simulink model "linear_closed_loop"  (R2025b)
settings: Solver=VariableStepAuto  StartTime=0.0  StopTime=200  RelTol=1e-3
undefined symbols (not defined in the file or in its folder): ra, rw, SATP
libraries: simulink_extras x2, cstblocks x1
settings Model: Creator=ruben  LastModifiedBy=flori

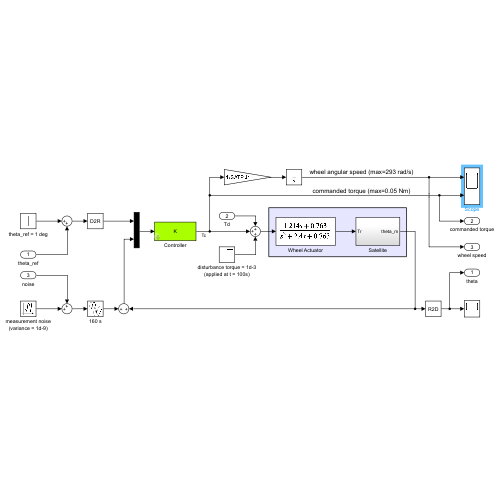
[thumbnail: Simulink's stored preview of the top-level diagram]
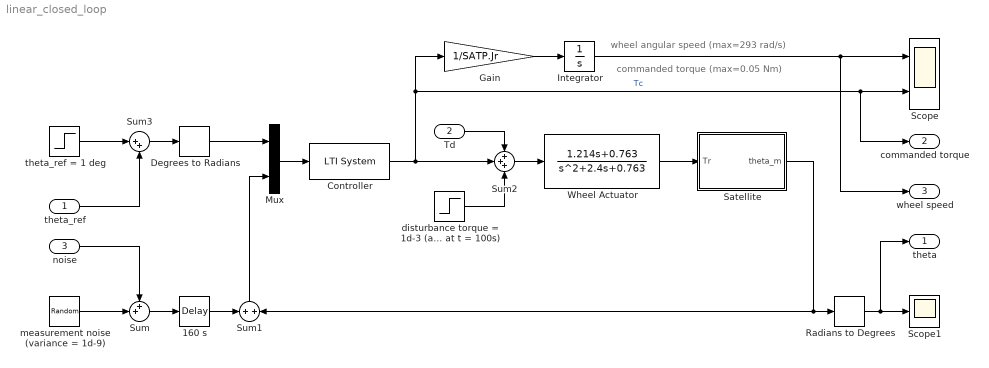
== system linear_closed_loop ==
  note: commanded torque (max=0.05 Nm)
  note: wheel angular speed (max=293 rad/s)
  theta_ref : Inport
  Td : Inport  Port=2
  noise : Inport  Port=3
  160 s : TransportDelay  DelayTime=160
  Controller : cstblocks/LTI System  sys=K  IC=[]  PadeOrder=0
  Degrees to Radians : simulink_extras/Transformations/Degrees to Radians
  Gain : Gain  Gain=1/SATP.Jr
  Integrator : Integrator
  Mux : Mux  Inputs=2
  Radians to Degrees : simulink_extras/Transformations/Radians to Degrees
  Satellite : Subsystem
  Scope : Scope  NumInputPorts=2
      settings: ActiveDisplayYMinimum=-302.85258313612223  ActiveDisplayYMaximum=227.5319246996597
  Scope1 : Scope
      settings: ActiveDisplayYMinimum=-0.33126841558150821  ActiveDisplayYMaximum=2.4578398850529664
  Sum : Sum  Inputs=++|
  Sum1 : Sum  Inputs=+|+
  Sum2 : Sum  Inputs=+++
  Sum3 : Sum  Inputs=|++
  Wheel Actuator : TransferFcn  Numerator=[1.214 0.763]  Denominator=[1 2.4 0.763]
  disturbance torque = 1d-3 (applied at t = 100s) : Step  Time=100  After=SATP.Td  SampleTime=0
  measurement noise (variance = 1d-9) : RandomNumber  Variance=SATP.sigmam2  SampleTime=0.01
  theta_ref = 1 deg : Step  Time=0  SampleTime=0
  theta : Outport
  commanded torque : Outport  Port=2
  wheel speed : Outport  Port=3
  wires:
  disturbance torque = 1d-3 (applied at t = 100s)/1 -> Sum2/3
  Sum/1 -> 160 s/1
  Sum2/1 -> Wheel Actuator/1
  measurement noise (variance = 1d-9)/1 -> Sum/2
  Gain/1 -> Integrator/1
  Mux/1 -> Controller/1
  Integrator/1 -> wheel speed/1, Scope/1
  theta_ref = 1 deg/1 -> Sum3/1
  noise/1 -> Sum/1
  theta_ref/1 -> Sum3/2
  160 s/1 -> Sum1/1
  Satellite/1(theta_m) -> Radians to Degrees/1, Sum1/2
  Radians to Degrees/1 -> Scope1/1, theta/1
  Degrees to Radians/1 -> Mux/1
  Td/1 -> Sum2/1
  Sum3/1 -> Degrees to Radians/1
  Sum1/1 -> Mux/2
  Controller/1 -> Sum2/2, Gain/1, Scope/2, commanded torque/1  "Tc"
  Wheel Actuator/1 -> Satellite/1(Tr)

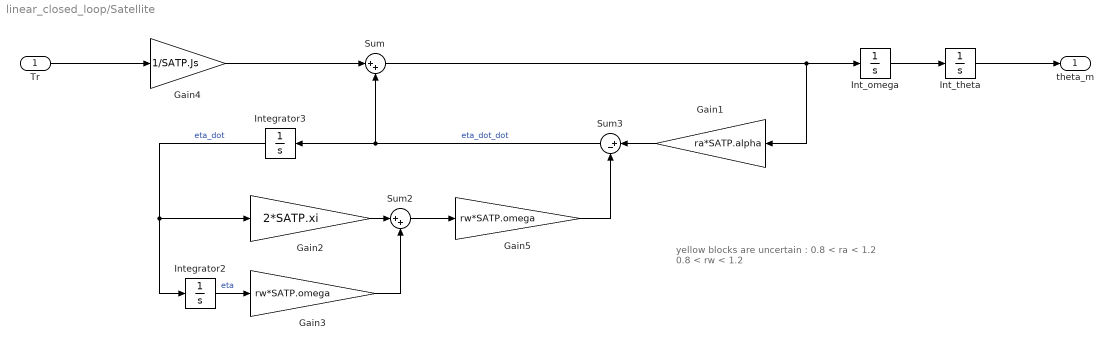
== system linear_closed_loop/Satellite ==
  note: yellow blocks are uncertain :
      | 0.8 < ra < 1.2
      | 0.8 < rw < 1.2
  Tr : Inport
  Gain1 : Gain  Gain=ra*SATP.alpha
  Gain2 : Gain  Gain=2*SATP.xi
  Gain3 : Gain  Gain=rw*SATP.omega
  Gain4 : Gain  Gain=1/SATP.Js
  Gain5 : Gain  Gain=rw*SATP.omega
  Int_omega : Integrator
  Int_theta : Integrator
  Integrator2 : Integrator  InitialCondition=SATP.eta0
  Integrator3 : Integrator
  Sum : Sum  Inputs=|++
  Sum2 : Sum  Inputs=|++
  Sum3 : Sum  Inputs=|+-
  theta_m : Outport
  wires:
  Integrator3/1 -> Integrator2/1, Gain2/1  "eta_dot"
  Int_omega/1 -> Int_theta/1
  Sum/1 -> Int_omega/1, Gain1/1
  Gain2/1 -> Sum2/1
  Gain4/1 -> Sum/1
  Gain3/1 -> Sum2/2
  Gain1/1 -> Sum3/1
  Tr/1 -> Gain4/1
  Sum3/1 -> Integrator3/1, Sum/2  "eta_dot_dot"
  Int_theta/1 -> theta_m/1
  Integrator2/1 -> Gain3/1  "eta"
  Sum2/1 -> Gain5/1
  Gain5/1 -> Sum3/2
